simulink model "Static_Target_Final_2a"  (R2020b)
settings: Solver=FixedStepDiscrete  StartTime=0.0  StopTime=60*2  FixedStep=dt  RelTol=1e-3
InitFcn:
  | close all
  | clear
  | clc
  | 
  | dtsim = 0.1;
  | dt =0.005;
  | dtdata = 0.01;
  | dtcontrol = 0.01;
  | 
  | % Enviromental Constants/System Parameters
  | 
  | mu = 398600; %km^3/s^2 (Earth)
  | 
  | I = [1.01560749 0.00028915 0.00002257;
  |        0.00028915 0.17343628 0.00936307;
  |        0.00002257 0.00936307 1.01561864];
  | 
  | I_inv =[1/I(1,1) 0 0; 0 1/I(2,2) 0; 0 0 1/I(3,3)];
  | 
  | % Inital Conditions
  | 
  | Y = 0;
  | P = 0;
  | R = 0;
  | 
  | a = 6378;
  | n = sqrt(mu/a^3);
  | 
  | wo = [0;0;0];
  | ho = [0;0;0];
  | 
  | % YPR to Quaternion
  | 
  | qo = [-cos(R/2)*sin(P/2)*sin(Y/2) + sin(R/2)*cos(P/2)*cos(Y/2);
  |           cos(R/2)*sin(P/2)*cos(Y/2) + sin(R/2)*cos(P/2)*sin(Y/2);
  |          -sin(R/2)*sin(P/2)*cos(Y/2) + cos(R/2)*cos(P/2)*sin(Y/2);
  |           sin(R/2)*sin(P/2)*sin(Y/2) + cos(R/2)*cos(P/2)*cos(Y/2)];
  | 
  | % Reaction Wheels
  | 
  | x = cosd(70);
  | y = sqrt(0.5*(1^2-x^2));
  | e1 = [x;y;y];
  | e2 = [x;-y;y];
  | e3 = [x;-y;-y];
  | e4 = [x;y;-y];
  | %e1 = [y;x;y];
  | %e2 = [-y;x;y];
  | %e3 = [-y;-x;y];
  | %e4 = [y;-x;y];
  | e = [e1 e2 e3 e4];
  | 
  | % Reaction Wheels MOI and Ang Vel
  | 
  | Irw = 0.000453158;
  | 
  | w1 =1500*2*pi/60;
  | w2 = 1500*2*pi/60;
  | w3 = -1500*2*pi/60;
  | w4 = -1500*2*pi/60;
  | 
  | alpha_max = 1537.9; %rad/sec^2 Look at picture
  | 
  | Tmax = Irw*alpha_max; % Irw*alpha_max;
  | 
  | %User Input
  | 
  | Yt = 90*pi/180;
  | Pt = 10*pi/180;
  | Rt = 30*pi/180;
  | 
  | YPRtarget = [Yt, Pt, Rt];
  | 
  | %User Input Check
  | 
  | if Pt > 20*pi/180
  | 
  | error('Input a pitch angle lower that 20 degrees')
  | 
  | end
  | 
  | q_target = [-cos(Rt/2)*sin(Pt/2)*sin(Yt/2) + sin(Rt/2)*cos(Pt/2)*cos(Yt/2);
  |                   cos(Rt/2)*sin(Pt/2)*cos(Yt/2) + sin(Rt/2)*cos(Pt/2)*sin(Yt/2);
  |                  -sin(Rt/2)*sin(Pt/2)*cos(Yt/2) + cos(Rt/2)*cos(Pt/2)*sin(Yt/2);
  |                   sin(Rt/2)*sin(Pt/2)*sin(Yt/2) + cos(Rt/2)*cos(Pt/2)*cos(Yt/2)];
  | 
  | %LQR Controller
  | 
  | k1 = (I(2,2) - I(3,3))/I(1,1);
  | k2 = (I(2,2) - I(3,3))/I(2,2);
  | k3 = (I(2,2) - I(1,1))/I(3,3);
  | 
  | F = -2*n^2*[4*k1, 0, 0;0, 3*k2, 0; 0, 0, k3];
  | G = n*[0 0 (1-k1);0 0 0;(k3-1) 0 0 ];
  | 
  | A = [zeros(3,3) 0.5*eye(3);F G];
  | B = [zeros(3,3); I_inv];
  | R = eye(3);
  | R_inv = R^-1;
  | 
  | Q_nominal= diag([1,1,1,10,10,10]);
  | S_nominal = icare(A,B,Q_nominal,R);
  | K_nominal = -R_inv*B'*S_nominal;
  | 
  | Q_corrective= diag([1,1,1,10,10,10]);
  | S_corrective = icare(A,B,Q_corrective,R);
  | K_corrective = -R_inv*B'*S_corrective;
  | 
  | Q_yawsweep= diag([1,1,1,10,15,10]);
  | S_yawsweep = icare(A,B,Q_yawsweep,R);
  | K_yawsweep = -R_inv*B'*S_yawsweep;
  | 
  | % Visual Int
  | 
  | myworld = vrworld('SimulinkTest.wrl');
  | open(myworld);
  | 
  | set(0,'Units','pixels');
  | scnsize = get(0,'ScreenSize');
  | 
  | f1 = vrfigure(myworld,scnsize);
StopFcn:
  | close all
  | 
  | %Set default grid axes to be on
  | set(groot,'defaultAxesXGrid','on')
  | set(groot,'defaultAxesYGrid','on')
  | 
  | 
  | %Create YPR subplots
  | figure(1)
  | subplot(1,3,1)
  | movegui('northeast')
  | plot(YPR.time,YPR.signals.values(:,1)*180/pi,'-k')
  | hold on
  | plot([0 YPR.time(end)], [1,1]*(rad2deg(YPRtarget(1))+1),'-r')
  | plot([0 YPR.time(end)], [1,1]*(rad2deg(YPRtarget(1))-1),'-r')
  | xlabel('Time (s)')
  | ylabel('Roll (deg)')
  | xlim([0 YPR.time(end)])
  | 
  | set(gca, 'FontSize', 15)
  | 
  | subplot(1,3,2)
  | plot(YPR.time,YPR.signals.values(:,2)*180/pi,'-k')
  | hold on
  | plot([0 YPR.time(end)],  [1,1]*(rad2deg(YPRtarget(2))+1),'-r')
  | plot([0 YPR.time(end)], [1,1]*(rad2deg(YPRtarget(2))-1),'-r')
  | xlabel('Time (s)')
  | ylabel('Pitch (deg)')
  | xlim([0 YPR.time(end)])
  | 
  | set(gca, 'FontSize', 15)
  | 
  | subplot(1,3,3)
  | plot(YPR.time,YPR.signals.values(:,3)*180/pi,'-k')
  | hold on
  | plot([0 YPR.time(end)],  [1,1]*(rad2deg(YPRtarget(3))+1),'-r')
  | plot([0 YPR.time(end)], [1,1]*(rad2deg(YPRtarget(3))-1),'-r')
  | xlabel('Time (s)')
  | ylabel('Yaw (deg)')
  | xlim([0 YPR.time(end)])
  | 
  | set(gca, 'FontSize', 15)
  | 
  | 
  | %Create Angular Position Plots
  | 
  | MagnitudeAngle = 2*acos(q_target(1))*180/pi;
  | 
  | figure(2)
  | movegui('northwest')
  | 
  | hold on
  | 
  | plot(YPR.time,YPR_Mag,'-k')
  | plot([0 YPR.time(end)],  [1,1]*(MagnitudeAngle+1),'-r')
  | plot([0 YPR.time(end)], [1,1]*(MagnitudeAngle-1),'-r')
  | xlabel('Time (sec)')
  | ylabel('Angle (deg)')
  | xlim([0 YPR.time(end)])
  | title('Angular Position Magnitude')
  | box on
  | 
  | 
  | % Create Motor Torque plot
  | figure(3)
  | movegui('south')
  | 
  | %plot(YPR.time,(Motor_Torques.signals.values(1,:)/Tmax)*100,YPR.time,(Motor_Torques.signals.values(2,:)/Tmax)*100,YPR.time,(Motor_Torques.signals.values(3,:)/Tmax)*100,YPR.time,(Motor_Torques.signals.values(4,:)/Tmax)*100)
  | plot(YPR.time,Motor_Torques.signals.values(1,:),YPR.time,Motor_Torques.signals.values(2,:),YPR.time,Motor_Torques.signals.values(3,:),YPR.time,Motor_Torques.signals.values(4,:))
  | xlabel('Time (s)')
  | %ylabel('Torque Percentage (%)')
  | ylabel('Torque (Nm)')
  | title('Motor Torques')
  | legend('Top Motor','Right Motor','Left Motor','Bottom Motor')
  | 
  | 
  | %Create Angular Speed plot
  | figure(4)
  | movegui('southwest')
  | 
  | wmag = sqrt(wvec.signals.values(1,:).^2+wvec.signals.values(2,:).^2+wvec.signals.values(3,:).^2)*180/pi;
  | hold on
  | plot(YPR.time,wmag)
  | plot(YPR.time,0.25.*ones(numel(YPR.time),1))
  | %plot(YPR.time,60*ones(numel(YPR.time),1))
  | xlabel('Time (s)')
  | ylabel('Angular Speed (deg/s)')
  | ylim([-0.5, 20])
  | xlim([0 YPR.time(end)])
  | title('Angular Speed Magnitude')
  | legend('System Angluar Speed', '0.25 deg/s')
  | grid on
  | 
  | 
  | %Create YPR Error plot
  | figure(5)
  | movegui('southeast')
  | hold on
  | plot(YPRerror.time(:,1)', YPRerror.signals.values(:,1), YPRerror.time(:,1)', YPRerror.signals.values(:,2), YPRerror.time(:,1)', YPRerror.signals.values(:,3))
  | plot(YPRerror.time(:,1)', zeros(length(YPRerror.time),1), '--')
  | xlabel('Time (s)')
  | ylabel('Error (°)')
  | title('YPR Error')
  | legend('Roll Error', 'Pitch Error', 'Yaw Error', 'Zero Error')
  | 
  | 
  | %Create Controller Type plot
  | figure(6)
  | movegui('north')
  | 
  | plot(controllerMode.time(:,1)', controllerMode.signals.values)
  | xlabel('Time (s)')
  | ylabel('Controller ID Tag')
  | title('LQR Control Mode vs Time')
  | ylim([0 4])
  | yticks([1,2,3])
undefined symbols (not defined in the file): DiscIntNeverNeededParam
libraries: vrlib x2, dspinverses x1, simulink x1
settings Model: Creator=lewisbreslin  LastModifiedBy=bnich
settings DataIOCC: ReturnWorkspaceOutputs=off
settings DebuggingCC: ArithmeticOperatorsInVariantConditions=warning
settings SFSimCC: SimUseLocalCustomCode=off  CustomCodeUndefinedFunction=UseInterfaceOnly
settings RTWCC: RTWUseLocalCustomCode=off
settings CodeAppCC: StateflowObjectComments=on

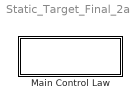
== system Static_Target_Final_2a ==
  "Main Control Law " : Subsystem  TreatAsAtomicUnit=on

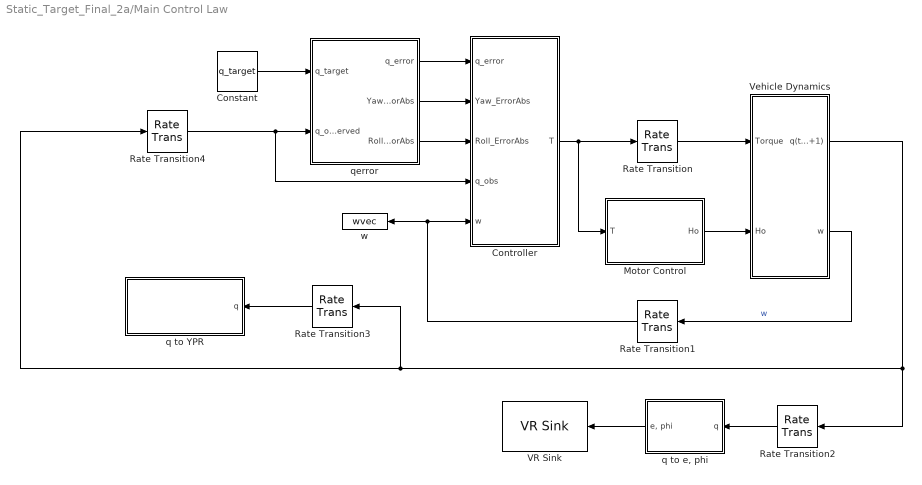
== system Static_Target_Final_2a/Main Control Law  ==
  Constant : Constant  Value=q_target
  Controller : Subsystem
  Motor Control : Subsystem
  Rate Transition : RateTransition  OutPortSampleTime=dt
  Rate Transition1 : RateTransition  InitialCondition=wo  OutPortSampleTime=dtcontrol
  Rate Transition2 : RateTransition  InitialCondition=qo  OutPortSampleTime=dtsim
  Rate Transition3 : RateTransition  InitialCondition=qo  OutPortSampleTime=dtdata
  Rate Transition4 : RateTransition  InitialCondition=qo  OutPortSampleTime=dtcontrol
  VR Sink : vrlib/VR Sink  InstantiateOnLoad=on  SampleTime=0.1  ViewEnable=on  RemoteChange=off  RemoteView=off  FieldsWritten=Phoenix.rotation.4.1.1.double  WorldFileName=SimulinkTest.wrl  AutoView=off  VideoDimensions=[]  AllowVariableSize=off
  Vehicle Dynamics : Subsystem
  q to YPR : Subsystem  TreatAsAtomicUnit=on
  "q to e, phi " : Subsystem
  qerror : Subsystem
  "w " : ToWorkspace  VariableName=wvec  SaveFormat=Structure With Time  SampleTime=-1
  wires:
  Vehicle Dynamics/2(w) -> Rate Transition1/1  "w"
  Controller/1(T) -> Rate Transition/1, Motor Control/1(T)
  Motor Control/1(Ho) -> Vehicle Dynamics/2("Ho ")
  qerror/3(Roll_ErrorAbs) -> Controller/3(Roll_ErrorAbs)
  Rate Transition3/1 -> q to YPR/1(q)
  qerror/2(Yaw_ErrorAbs) -> Controller/2(Yaw_ErrorAbs)
  qerror/1(q_error) -> Controller/1(q_error)
  Rate Transition2/1 -> "q to e, phi "/1(q)
  Constant/1 -> qerror/1(q_target)
  Rate Transition1/1 -> Controller/5(w), "w "/1
  Vehicle Dynamics/1(q(t_k+1)) -> Rate Transition2/1, Rate Transition4/1, Rate Transition3/1
  Rate Transition/1 -> Vehicle Dynamics/1(Torque)
  Rate Transition4/1 -> Controller/4(q_obs), qerror/2(q_observed)
  "q to e, phi "/1("e, phi") -> VR Sink/1

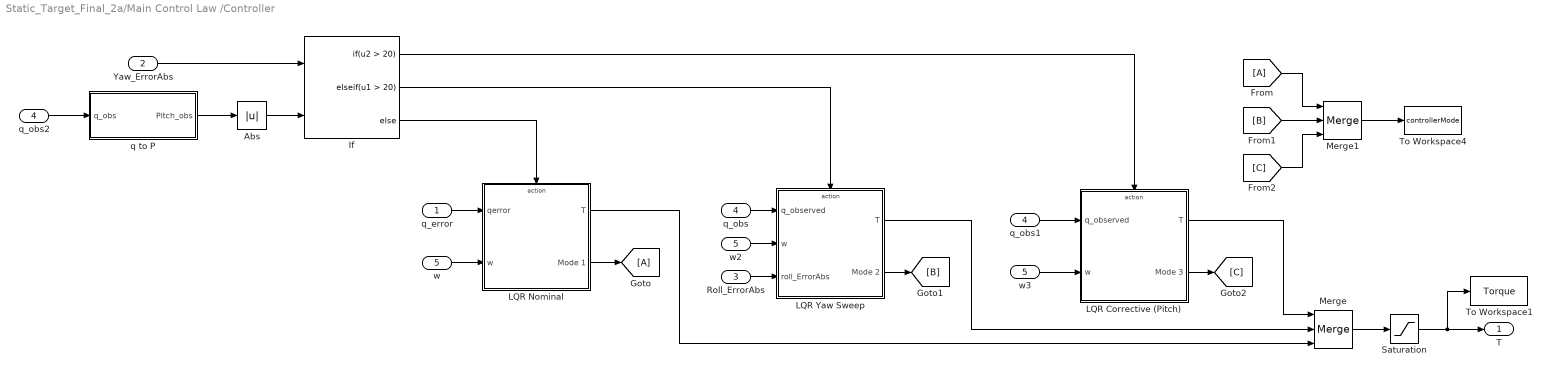
== system Static_Target_Final_2a/Main Control Law /Controller ==
  q_error : Inport
  Yaw_ErrorAbs : Inport  Port=2
  Roll_ErrorAbs : Inport  Port=3
  q_obs : Inport  Port=4
  w : Inport  Port=5
  Abs : Abs
  If : If  NumInputs=2  IfExpression=u2 > 20  ElseIfExpressions=u1 > 20
  LQR Corrective (Pitch) : Subsystem
  LQR Nominal : Subsystem  TreatAsAtomicUnit=on
  LQR Yaw Sweep : Subsystem
  Merge : Merge  Inputs=3
  Merge1 : Merge  Inputs=3
  Saturation : Saturate  UpperLimit=Tmax  LowerLimit=-Tmax
  To Workspace1 : ToWorkspace  VariableName=Torque  SaveFormat=Structure With Time  SampleTime=-1
  To Workspace4 : ToWorkspace  VariableName=controllerMode  SaveFormat=Structure With Time  SampleTime=-1
  q to P : Subsystem
  q_obs1 : InportShadow  Port=4
  q_obs2 : InportShadow  Port=4
  w2 : InportShadow  Port=5
  w3 : InportShadow  Port=5
  T : Outport
  wires:
  Yaw_ErrorAbs/1 -> If/1
  If/3 -> LQR Nominal/Action
  q_error/1 -> LQR Nominal/1(qerror)
  If/1 -> LQR Corrective (Pitch)/Action
  q_obs1/1 -> LQR Corrective (Pitch)/1(q_observed)
  q_obs/1 -> LQR Yaw Sweep/1(q_observed)
  q to P/1(Pitch_obs) -> Abs/1
  If/2 -> LQR Yaw Sweep/Action
  LQR Nominal/2(Mode 1) -> [A]
  LQR Yaw Sweep/2(Mode 2) -> [B]
  LQR Corrective (Pitch)/2(Mode 3) -> [C]
  [B] -> Merge1/2
  [A] -> Merge1/1
  [C] -> Merge1/3
  Merge1/1 -> To Workspace4/1
  w3/1 -> LQR Corrective (Pitch)/2(w)
  w2/1 -> LQR Yaw Sweep/2(w)
  w/1 -> LQR Nominal/2(w)
  q_obs2/1 -> q to P/1(q_obs)
  Abs/1 -> If/2
  Roll_ErrorAbs/1 -> LQR Yaw Sweep/3(roll_ErrorAbs)
  LQR Nominal/1(T) -> Merge/3
  LQR Yaw Sweep/1(T) -> Merge/2
  LQR Corrective (Pitch)/1(T) -> Merge/1
  Merge/1 -> Saturation/1
  Saturation/1 -> To Workspace1/1, T/1

== system Static_Target_Final_2a/Main Control Law /Motor Control ==
  T : Inport
  Actuator : Subsystem
  Motor control : Subsystem
  Ho : Outport
  wires:
  T/1 -> Actuator/1(Torque)
  Actuator/2(alpha_RW) -> Motor control/2(alpha_RW)
  Motor control/1(Ho) -> Ho/1
  Actuator/1(Irw*e) -> Motor control/1(Irw*e)

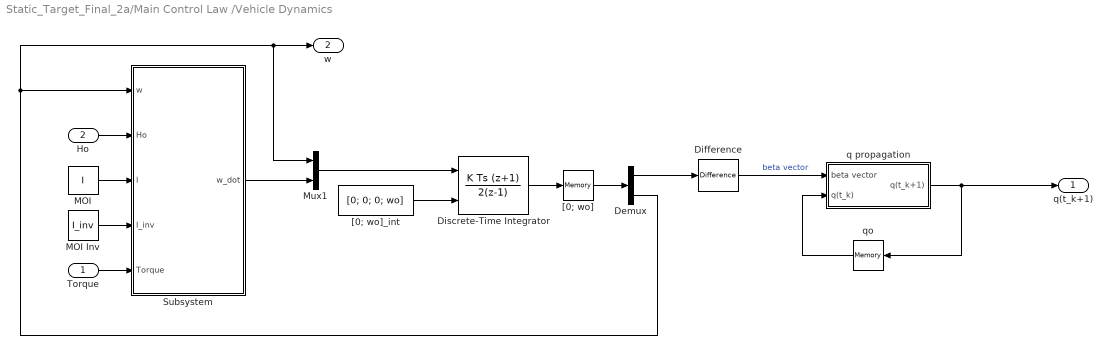
== system Static_Target_Final_2a/Main Control Law /Vehicle Dynamics ==
  Torque : Inport
  "Ho " : Inport  Port=2
  Demux : Demux  Outputs=2
  Difference : simulink/Discrete/Difference  ICPrevInput=[0;0;0]  OutMin=[]  OutMax=[]  OutDataType=fixdt(1, 16)  OutScaling=2^-10  DoSatur=off
  Discrete-Time Integrator : DiscreteIntegrator  IntegratorMethod=Integration: Trapezoidal  InitialConditionSource=external  SampleTime=dt  ICPrevOutput=DiscIntNeverNeededParam  ICPrevScaledInput=DiscIntNeverNeededParam
  MOI : Constant  Value=I
  MOI Inv : Constant  Value=I_inv
  Mux1 : Mux  Inputs=2
  Subsystem : Subsystem
  "[0; wo]" : Memory  InitialCondition=[0;0;0;wo]  InheritSampleTime=on
  "[0; wo]_int" : Constant  Value=[0; 0; 0; wo]  VectorParams1D=off  SampleTime=dt
  q propagation : Subsystem
  qo : Memory  InitialCondition=qo  InheritSampleTime=on
  q(t_k+1) : Outport
  w : Outport  Port=2
  wires:
  "Ho "/1 -> Subsystem/2("Ho ")
  Torque/1 -> Subsystem/5(Torque)
  MOI Inv/1 -> Subsystem/4(I_inv)
  MOI/1 -> Subsystem/3(I)
  Subsystem/1(w_dot) -> Mux1/2
  Difference/1 -> q propagation/1("beta vector ")  "beta vector"
  "[0; wo]_int"/1 -> Discrete-Time Integrator/2
  q propagation/1(q(t_k+1)) -> q(t_k+1)/1, qo/1
  qo/1 -> q propagation/2(q(t_k))
  Demux/1 -> Difference/1
  Discrete-Time Integrator/1 -> "[0; wo]"/1
  "[0; wo]"/1 -> Demux/1
  Mux1/1 -> Discrete-Time Integrator/1
  Demux/2 -> w/1, Mux1/1, Subsystem/1(w)

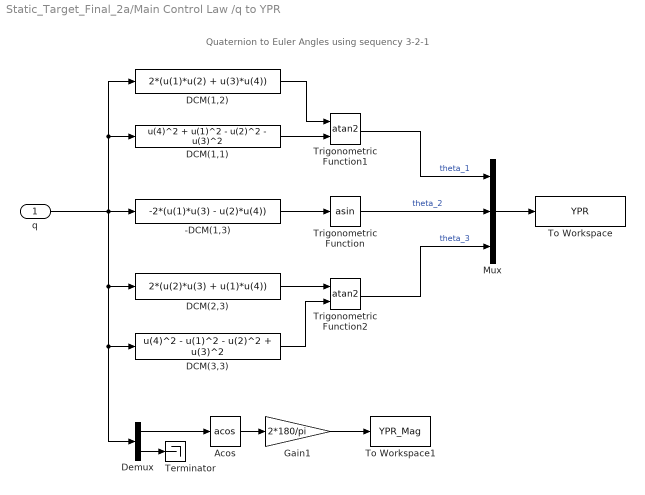
== system Static_Target_Final_2a/Main Control Law /q to YPR ==
  note: Quaternion to Euler Angles using sequency 3-2-1
  q : Inport
  -DCM(1,3) : Fcn  Expr=-2*(u(1)*u(3) - u(2)*u(4))
  Acos : Trigonometry  Operator=acos
  DCM(1,1) : Fcn  Expr=u(4)^2 + u(1)^2 - u(2)^2 - u(3)^2
  DCM(1,2) : Fcn  Expr=2*(u(1)*u(2) + u(3)*u(4))
  DCM(2,3) : Fcn  Expr=2*(u(2)*u(3) + u(1)*u(4))
  DCM(3,3) : Fcn  Expr=u(4)^2 - u(1)^2 - u(2)^2 + u(3)^2
  Demux : Demux  Outputs=[1;3]
  Gain1 : Gain  Gain=2*180/pi
  Mux : Mux  Inputs=3
  Terminator : Terminator
  To Workspace : ToWorkspace  VariableName=YPR  SaveFormat=Structure With Time  SampleTime=dtdata
  To Workspace1 : ToWorkspace  VariableName=YPR_Mag  SampleTime=dtdata
  Trigonometric Function : Trigonometry  Operator=asin
  Trigonometric Function1 : Trigonometry  Operator=atan2
  Trigonometric Function2 : Trigonometry  Operator=atan2
  wires:
  q/1 -> Demux/1, DCM(3,3)/1, DCM(2,3)/1, -DCM(1,3)/1, DCM(1,2)/1, DCM(1,1)/1
  -DCM(1,3)/1 -> Trigonometric Function/1
  DCM(2,3)/1 -> Trigonometric Function2/1
  DCM(1,2)/1 -> Trigonometric Function1/1
  DCM(1,1)/1 -> Trigonometric Function1/2
  DCM(3,3)/1 -> Trigonometric Function2/2
  Trigonometric Function/1 -> Mux/2  "theta_2"
  Trigonometric Function2/1 -> Mux/3  "theta_3"
  Trigonometric Function1/1 -> Mux/1  "theta_1"
  Mux/1 -> To Workspace/1
  Gain1/1 -> To Workspace1/1
  Acos/1 -> Gain1/1
  Demux/1 -> Acos/1
  Demux/2 -> Terminator/1

== system Static_Target_Final_2a/Main Control Law /q to e, phi  ==
  note: Quaternion to Euler Angles using sequency 3-2-1
  q : Inport
  Demux : Demux  Outputs=[3, 1]
  Divide : Product  Inputs=*/
  Gain : Gain  Gain=2
  Mux : Mux  Inputs=2
  Trigonometric Function : Trigonometry  Operator=acos
  Trigonometric Function1 : Trigonometry
  "e, phi" : Outport
  wires:
  Gain/1 -> Mux/2  "phi"
  Demux/2 -> Trigonometric Function/1  "q4"
  Trigonometric Function/1 -> Gain/1, Trigonometric Function1/1  "phi/2"
  Demux/1 -> Divide/1  "q_hat"
  Divide/1 -> Mux/1  "e"
  Trigonometric Function1/1 -> Divide/2  "sin(phi/2)"
  Mux/1 -> "e, phi"/1
  q/1 -> Demux/1

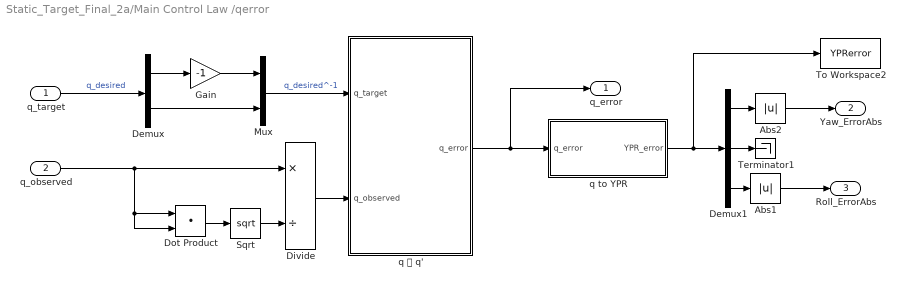
== system Static_Target_Final_2a/Main Control Law /qerror ==
  q_target : Inport
  q_observed : Inport  Port=2
  Abs1 : Abs
  Abs2 : Abs
  Demux : Demux  Outputs=[3,1]
  Demux1 : Demux  Outputs=3
  Divide : Product  Inputs=*/
  Dot Product : DotProduct  InputSameDT=on  OutDataTypeStr=Inherit: Inherit via internal rule
  Gain : Gain  Gain=-1
  Mux : Mux  Inputs=2
  Sqrt : Sqrt  SaturateOnIntegerOverflow=on
  Terminator1 : Terminator
  To Workspace2 : ToWorkspace  VariableName=YPRerror  SaveFormat=Structure With Time  SampleTime=-1
  q to YPR : Subsystem  TreatAsAtomicUnit=on
  q ⦻ q' : Subsystem  TreatAsAtomicUnit=on
  q_error : Outport
  Yaw_ErrorAbs : Outport  Port=2
  Roll_ErrorAbs : Outport  Port=3
  wires:
  Abs2/1 -> Yaw_ErrorAbs/1
  Demux1/2 -> Terminator1/1
  Abs1/1 -> Roll_ErrorAbs/1
  Divide/1 -> q ⦻ q'/2(q_observed)
  q_observed/1 -> Divide/1, Dot Product/1, Dot Product/2
  Dot Product/1 -> Sqrt/1
  q ⦻ q'/1(q_error) -> q to YPR/1(q_error), q_error/1
  Gain/1 -> Mux/1
  Mux/1 -> q ⦻ q'/1(q_target)  "q_desired^-1"
  q_target/1 -> Demux/1  "q_desired"
  Demux/1 -> Gain/1
  Sqrt/1 -> Divide/2
  Demux/2 -> Mux/2
  q to YPR/1(YPR_error) -> Demux1/1, To Workspace2/1
  Demux1/1 -> Abs2/1
  Demux1/3 -> Abs1/1

== system Static_Target_Final_2a/Main Control Law /Controller/LQR Corrective (Pitch) ==
  q_observed : Inport
  w : Inport  Port=2
  Action Port : ActionPort  ActionPortLabel=if(u2 > 20)
  Constant : Constant  Value=3
  LQR Corrective (Pitch) : Subsystem
  q_adjustment : Subsystem
  q_error : Subsystem
  T : Outport
  Mode 3 : Outport  Port=2
  wires:
  Constant/1 -> Mode 3/1
  LQR Corrective (Pitch)/1(T) -> T/1
  w/1 -> LQR Corrective (Pitch)/2(w)
  q_adjustment/1(q_adjusted) -> q_error/1(q_target)
  q_observed/1 -> q_adjustment/1(q_obs), q_error/2(q_observed)
  q_error/1(q_error) -> LQR Corrective (Pitch)/1(q_error)

== system Static_Target_Final_2a/Main Control Law /Controller/LQR Nominal ==
  qerror : Inport
  w : Inport  Port=2
  Action Port : ActionPort  ActionPortLabel=else
  Constant : Constant
  LQR Nominal : Subsystem
  T : Outport
  Mode 1 : Outport  Port=2
  wires:
  Constant/1 -> Mode 1/1
  qerror/1 -> LQR Nominal/1(q_error)
  LQR Nominal/1(T) -> T/1
  w/1 -> LQR Nominal/2(w)

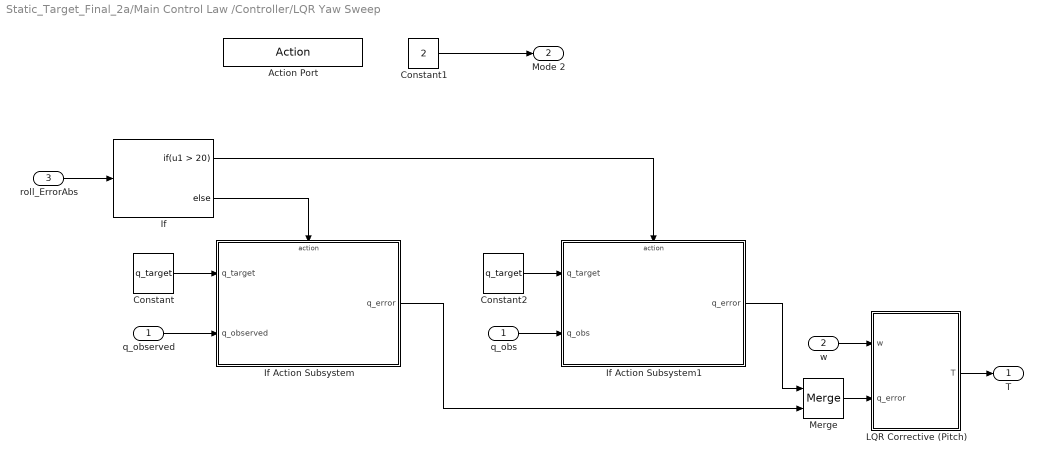
== system Static_Target_Final_2a/Main Control Law /Controller/LQR Yaw Sweep ==
  q_observed : Inport
  w : Inport  Port=2
  roll_ErrorAbs : Inport  Port=3
  Action Port : ActionPort  ActionPortLabel=elseif(u1 > 20)
  Constant : Constant  Value=q_target
  Constant1 : Constant  Value=2
  Constant2 : Constant  Value=q_target
  If : If  IfExpression=u1 > 20
  If Action Subsystem : Subsystem  TreatAsAtomicUnit=on
  If Action Subsystem1 : Subsystem  TreatAsAtomicUnit=on
  LQR Corrective (Pitch) : Subsystem
  Merge : Merge
  q_obs : InportShadow
  T : Outport
  Mode 2 : Outport  Port=2
  wires:
  roll_ErrorAbs/1 -> If/1
  Constant/1 -> If Action Subsystem/1(q_target)
  Constant1/1 -> Mode 2/1
  If/2 -> If Action Subsystem/Action
  LQR Corrective (Pitch)/1(T) -> T/1
  w/1 -> LQR Corrective (Pitch)/1(w)
  If/1 -> If Action Subsystem1/Action
  q_observed/1 -> If Action Subsystem/2(q_observed)
  Merge/1 -> LQR Corrective (Pitch)/2(q_error)
  If Action Subsystem1/1(q_error) -> Merge/1
  If Action Subsystem/1(q_error) -> Merge/2
  q_obs/1 -> If Action Subsystem1/2(q_obs)
  Constant2/1 -> If Action Subsystem1/1(q_target)

== system Static_Target_Final_2a/Main Control Law /Controller/q to P ==
  q_obs : Inport
  -DCM(1,3) : Fcn  Expr=-2*(u(1)*u(3) - u(2)*u(4))
  Gain2 : Gain  Gain=180/pi
  Trigonometric Function1 : Trigonometry  Operator=asin
  Pitch_obs : Outport
  wires:
  Gain2/1 -> Pitch_obs/1
  Trigonometric Function1/1 -> Gain2/1  "P"
  -DCM(1,3)/1 -> Trigonometric Function1/1
  q_obs/1 -> -DCM(1,3)/1

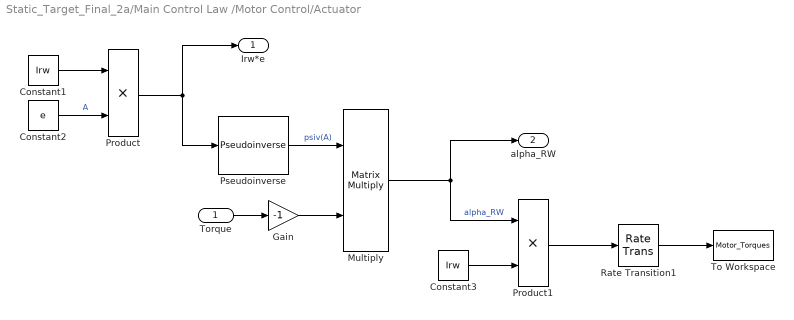
== system Static_Target_Final_2a/Main Control Law /Motor Control/Actuator ==
  Torque : Inport  PortDimensions=[3,1]
  Constant1 : Constant  Value=Irw
  Constant2 : Constant  Value=e
  Constant3 : Constant  Value=Irw
  Gain : Gain  Gain=-1
  Multiply : Product  Multiplication=Matrix(*)
  Product : Product
  Product1 : Product
  Pseudoinverse : dspinverses/Pseudoinverse  wanterr=off  SimulateUsing=Interpreted execution
      settings: SourceProductBaseCode=DS
  Rate Transition1 : RateTransition  InitialCondition=[0;0;0;0]  OutPortSampleTime=dtdata
  To Workspace : ToWorkspace  VariableName=Motor_Torques  SaveFormat=Structure With Time  SampleTime=dtdata
  Irw*e : Outport
  alpha_RW : Outport  Port=2
  wires:
  Torque/1 -> Gain/1
  Product/1 -> Irw*e/1, Pseudoinverse/1
  Constant1/1 -> Product/1
  Pseudoinverse/1 -> Multiply/1  "psiv(A)"
  Multiply/1 -> Product1/1, alpha_RW/1  "alpha_RW"
  Constant2/1 -> Product/2  "A"
  Gain/1 -> Multiply/2
  Constant3/1 -> Product1/2
  Product1/1 -> Rate Transition1/1
  Rate Transition1/1 -> To Workspace/1

== system Static_Target_Final_2a/Main Control Law /Motor Control/Motor control ==
  Irw*e : Inport
  alpha_RW : Inport  Port=2
  Constant3 : Constant  Value=[w1 ;w2 ;w3 ;w4]  SampleTime=dt
  Discrete-Time Integrator1 : DiscreteIntegrator  IntegratorMethod=Integration: Trapezoidal  InitialConditionSource=external  SampleTime=dt  LimitOutput=on  UpperSaturationLimit=733  LowerSaturationLimit=-733  ICPrevOutput=DiscIntNeverNeededParam  ICPrevScaledInput=DiscIntNeverNeededParam
  Multiply3 : Product  Multiplication=Matrix(*)
  Ho : Outport
  wires:
  Irw*e/1 -> Multiply3/1  "Irw*e"
  Constant3/1 -> Discrete-Time Integrator1/2
  Multiply3/1 -> Ho/1
  Discrete-Time Integrator1/1 -> Multiply3/2
  alpha_RW/1 -> Discrete-Time Integrator1/1

== system Static_Target_Final_2a/Main Control Law /Vehicle Dynamics/Subsystem ==
  note: $\dot{\bar{\omega}}=[I]^{-1}\left(\bar{T}-\bar{\omega} \times\left([I]\bar{\omega}+\bar{H_0}\right)\right)$
  w : Inport
  "Ho " : Inport  Port=2
  I : Inport  Port=3
  I_inv : Inport  Port=4
  Torque : Inport  Port=5
  Add1 : Sum  Inputs=|++
  Cross Product : vrlib/Utilities/Cross Product
  Matrix Multiply2 : Product  Multiplication=Matrix(*)
  Matrix Multiply3 : Product  Multiplication=Matrix(*)
  Sum : Sum  Inputs=|+-
  w_dot : Outport
  wires:
  I/1 -> Matrix Multiply2/1
  w/1 -> Cross Product/1, Matrix Multiply2/2
  Torque/1 -> Sum/1
  Sum/1 -> Matrix Multiply3/2
  Cross Product/1 -> Sum/2
  Matrix Multiply3/1 -> w_dot/1
  I_inv/1 -> Matrix Multiply3/1
  Matrix Multiply2/1 -> Add1/1
  Add1/1 -> Cross Product/2
  "Ho "/1 -> Add1/2

== system Static_Target_Final_2a/Main Control Law /Vehicle Dynamics/q propagation ==
  "beta vector " : Inport
  q(t_k) : Inport  Port=2
  Dot Product : DotProduct  InputSameDT=on  OutDataTypeStr=Inherit: Inherit via internal rule
  Sqrt : Sqrt  SaturateOnIntegerOverflow=on
  if/esle condition : Subsystem
  q * q' : Subsystem  TreatAsAtomicUnit=on
  q(t_k+1) : Outport
  wires:
  "beta vector "/1 -> Dot Product/2, Dot Product/1, if/esle condition/1("beta vector ")
  if/esle condition/1(q') -> q * q'/2(q')
  q(t_k)/1 -> q * q'/1(q)
  q * q'/1(q'') -> q(t_k+1)/1
  Dot Product/1 -> Sqrt/1
  Sqrt/1 -> if/esle condition/2(norm(beta))

== system Static_Target_Final_2a/Main Control Law /qerror/q to YPR ==
  note: Quaternion to Euler Angles using sequency 3-2-1
  q_error : Inport
  -DCM(1,3) : Fcn  Expr=-2*(u(1)*u(3) - u(2)*u(4))
  DCM(1,1) : Fcn  Expr=u(4)^2 + u(1)^2 - u(2)^2 - u(3)^2
  DCM(1,2) : Fcn  Expr=2*(u(1)*u(2) + u(3)*u(4))
  DCM(2,3) : Fcn  Expr=2*(u(2)*u(3) + u(1)*u(4))
  DCM(3,3) : Fcn  Expr=u(4)^2 - u(1)^2 - u(2)^2 + u(3)^2
  Gain2 : Gain  Gain=180/pi
  Mux : Mux  Inputs=3
  Trigonometric Function : Trigonometry  Operator=asin
  Trigonometric Function1 : Trigonometry  Operator=atan2
  Trigonometric Function2 : Trigonometry  Operator=atan2
  YPR_error : Outport
  wires:
  q_error/1 -> DCM(3,3)/1, DCM(2,3)/1, -DCM(1,3)/1, DCM(1,2)/1, DCM(1,1)/1
  -DCM(1,3)/1 -> Trigonometric Function/1
  DCM(2,3)/1 -> Trigonometric Function2/1
  DCM(1,2)/1 -> Trigonometric Function1/1
  DCM(1,1)/1 -> Trigonometric Function1/2
  DCM(3,3)/1 -> Trigonometric Function2/2
  Trigonometric Function/1 -> Mux/2  "P"
  Trigonometric Function2/1 -> Mux/3  "R"
  Trigonometric Function1/1 -> Mux/1  "Y"
  Gain2/1 -> YPR_error/1
  Mux/1 -> Gain2/1

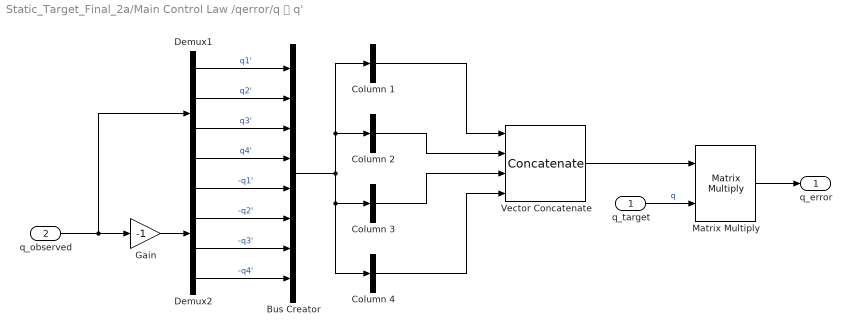
== system Static_Target_Final_2a/Main Control Law /qerror/q ⦻ q' ==
  q_target : Inport
  q_observed : Inport  Port=2
  Bus Creator : BusCreator  Inputs=8
  Column 1 : BusSelector  OutputSignals=q4',-q3',q2',-q1'  OutputAsBus=on
  Column 2 : BusSelector  OutputSignals=q3',q4',-q1',-q2'  OutputAsBus=on
  Column 3 : BusSelector  OutputSignals=-q2',q1',q4',-q3'  OutputAsBus=on
  Column 4 : BusSelector  OutputSignals=q1',q2',q3',q4'  OutputAsBus=on
  Demux1 : Demux
  Demux2 : Demux
  Gain : Gain  Gain=-1
  Matrix Multiply : Product  Multiplication=Matrix(*)
  Vector Concatenate : Concatenate  NumInputs=4  Mode=Multidimensional array  ConcatenateDimension=2
  q_error : Outport
  wires:
  Gain/1 -> Demux2/1
  Demux1/1 -> Bus Creator/1  "q1'"
  Demux1/3 -> Bus Creator/3  "q3'"
  Demux1/2 -> Bus Creator/2  "q2'"
  Demux2/4 -> Bus Creator/8  "-q4'"
  Demux2/3 -> Bus Creator/7  "-q3'"
  Demux2/2 -> Bus Creator/6  "-q2'"
  Demux2/1 -> Bus Creator/5  "-q1'"
  Demux1/4 -> Bus Creator/4  "q4'"
  Bus Creator/1 -> Column 4/1, Column 3/1, Column 1/1, Column 2/1
  Column 1/1 -> Vector Concatenate/1
  Column 2/1 -> Vector Concatenate/2
  Column 3/1 -> Vector Concatenate/3
  Column 4/1 -> Vector Concatenate/4
  q_observed/1 -> Demux1/1, Gain/1
  q_target/1 -> Matrix Multiply/2  "q"
  Matrix Multiply/1 -> q_error/1
  Vector Concatenate/1 -> Matrix Multiply/1

== system Static_Target_Final_2a/Main Control Law /Controller/LQR Corrective (Pitch)/LQR Corrective (Pitch) ==
  q_error : Inport
  w : Inport  Port=2
  Constant3 : Constant  Value=K_corrective
  Demux1 : Demux  Outputs=[3,1]
  Mux1 : Mux  Inputs=2
  Product : Product  Multiplication=Matrix(*)
  Terminator1 : Terminator
  T : Outport
  wires:
  Product/1 -> T/1
  q_error/1 -> Demux1/1
  Constant3/1 -> Product/1
  Demux1/1 -> Mux1/1  "qhat_Error"
  w/1 -> Mux1/2
  Mux1/1 -> Product/2  "xbar"
  Demux1/2 -> Terminator1/1

== system Static_Target_Final_2a/Main Control Law /Controller/LQR Corrective (Pitch)/q_adjustment ==
  q_obs : Inport
  DCM(1,1) : Fcn  Expr=u(4)^2 + u(1)^2 - u(2)^2 - u(3)^2
  DCM(1,2) : Fcn  Expr=2*(u(1)*u(2) + u(3)*u(4))
  DCM(2,3) : Fcn  Expr=2*(u(2)*u(3) + u(1)*u(4))
  DCM(3,3) : Fcn  Expr=u(4)^2 - u(1)^2 - u(2)^2 + u(3)^2
  Trigonometric Function4 : Trigonometry  Operator=atan2
  Trigonometric Function5 : Trigonometry  Operator=atan2
  YPR to q : Subsystem
  q_adjusted : Outport
  wires:
  Trigonometric Function5/1 -> YPR to q/2(R)  "R"
  DCM(2,3)/1 -> Trigonometric Function5/1
  DCM(1,1)/1 -> Trigonometric Function4/2
  DCM(3,3)/1 -> Trigonometric Function5/2
  DCM(1,2)/1 -> Trigonometric Function4/1
  q_obs/1 -> DCM(3,3)/1, DCM(2,3)/1, DCM(1,2)/1, DCM(1,1)/1
  YPR to q/1(q_adjusted) -> q_adjusted/1
  Trigonometric Function4/1 -> YPR to q/1(Y)  "Y"

== system Static_Target_Final_2a/Main Control Law /Controller/LQR Corrective (Pitch)/q_error ==
  q_target : Inport
  q_observed : Inport  Port=2
  Demux : Demux  Outputs=[3,1]
  Divide : Product  Inputs=*/
  Dot Product : DotProduct  InputSameDT=on  OutDataTypeStr=Inherit: Inherit via internal rule
  Gain : Gain  Gain=-1
  Mux : Mux  Inputs=2
  Sqrt : Sqrt  SaturateOnIntegerOverflow=on
  q ⦻ q' : Subsystem  TreatAsAtomicUnit=on
  q_error : Outport
  wires:
  q ⦻ q'/1(q_error) -> q_error/1
  Mux/1 -> q ⦻ q'/1(q_target)  "q_desired^-1"
  Sqrt/1 -> Divide/2
  Demux/1 -> Gain/1
  q_target/1 -> Demux/1  "q_desired"
  Gain/1 -> Mux/1
  q_observed/1 -> Divide/1, Dot Product/1, Dot Product/2
  Dot Product/1 -> Sqrt/1
  Demux/2 -> Mux/2
  Divide/1 -> q ⦻ q'/2(q_observed)

== system Static_Target_Final_2a/Main Control Law /Controller/LQR Nominal/LQR Nominal ==
  q_error : Inport
  w : Inport  Port=2
  Constant3 : Constant  Value=K_nominal
  Demux1 : Demux  Outputs=[3,1]
  Mux1 : Mux  Inputs=2
  Product : Product  Multiplication=Matrix(*)
  Terminator1 : Terminator
  T : Outport
  wires:
  Mux1/1 -> Product/2  "xbar"
  Demux1/1 -> Mux1/1  "qhat_Error"
  q_error/1 -> Demux1/1
  Demux1/2 -> Terminator1/1
  w/1 -> Mux1/2
  Constant3/1 -> Product/1
  Product/1 -> T/1

== system Static_Target_Final_2a/Main Control Law /Controller/LQR Yaw Sweep/If Action Subsystem ==
  q_target : Inport
  q_observed : Inport  Port=2
  Action Port : ActionPort  ActionPortLabel=else
  q_adjustment : Subsystem
  qerror : Subsystem
  q_error : Outport
  wires:
  q_target/1 -> q_adjustment/1(q_target)
  qerror/1(q_error) -> q_error/1
  q_observed/1 -> qerror/2(q_observed)
  q_adjustment/1(q_adjusted) -> qerror/1(q_target)

== system Static_Target_Final_2a/Main Control Law /Controller/LQR Yaw Sweep/If Action Subsystem1 ==
  q_target : Inport
  q_obs : Inport  Port=2
  Action Port : ActionPort  ActionPortLabel=if(u1 > 20)
  q_adjustment : Subsystem
  qerror : Subsystem
  q_error : Outport
  wires:
  q_adjustment/1(q_adjusted) -> qerror/1(q_target)
  q_target/1 -> q_adjustment/1(q_target)
  q_obs/1 -> qerror/2(q_observed), q_adjustment/2(q_obs)
  qerror/1(q_error) -> q_error/1

== system Static_Target_Final_2a/Main Control Law /Controller/LQR Yaw Sweep/LQR Corrective (Pitch) ==
  w : Inport
  q_error : Inport  Port=2
  Constant3 : Constant  Value=K_yawsweep
  Demux1 : Demux  Outputs=[3,1]
  Mux1 : Mux  Inputs=2
  Product : Product  Multiplication=Matrix(*)
  Terminator1 : Terminator
  T : Outport
  wires:
  Product/1 -> T/1
  q_error/1 -> Demux1/1
  Constant3/1 -> Product/1
  Demux1/1 -> Mux1/1  "qhat_Error"
  w/1 -> Mux1/2
  Mux1/1 -> Product/2  "xbar"
  Demux1/2 -> Terminator1/1

== system Static_Target_Final_2a/Main Control Law /Vehicle Dynamics/q propagation/if//esle condition ==
  "beta vector " : Inport
  norm(beta) : Inport  Port=2
  If : If  IfExpression=u1 < 1e-10
  If Action Subsystem : Subsystem  TreatAsAtomicUnit=on
  If Action Subsystem1 : Subsystem  TreatAsAtomicUnit=on
  Merge : Merge
  q' : Outport
  wires:
  If Action Subsystem/1(q') -> Merge/1
  Merge/1 -> q'/1
  If Action Subsystem1/1(q') -> Merge/2
  If/2 -> If Action Subsystem1/Action
  norm(beta)/1 -> If Action Subsystem1/1(norm(beta)), If/1
  If/1 -> If Action Subsystem/Action
  "beta vector "/1 -> If Action Subsystem1/2("beta vector ")

== system Static_Target_Final_2a/Main Control Law /Vehicle Dynamics/q propagation/q * q' ==
  q : Inport
  q' : Inport  Port=2
  Bus Creator : BusCreator  Inputs=8
  Column 1 : BusSelector  OutputSignals=q4',-q3',q2',-q1'  OutputAsBus=on
  Column 2 : BusSelector  OutputSignals=q3',q4',-q1',-q2'  OutputAsBus=on
  Column 3 : BusSelector  OutputSignals=-q2',q1',q4',-q3'  OutputAsBus=on
  Column 4 : BusSelector  OutputSignals=q1',q2',q3',q4'  OutputAsBus=on
  Demux1 : Demux
  Demux2 : Demux
  Gain : Gain  Gain=-1
  Matrix Multiply : Product  Multiplication=Matrix(*)
  Vector Concatenate : Concatenate  NumInputs=4  Mode=Multidimensional array  ConcatenateDimension=2
  q'' : Outport
  wires:
  Gain/1 -> Demux2/1
  Demux1/1 -> Bus Creator/1  "q1'"
  Demux1/3 -> Bus Creator/3  "q3'"
  Demux1/2 -> Bus Creator/2  "q2'"
  Demux2/4 -> Bus Creator/8  "-q4'"
  Demux2/3 -> Bus Creator/7  "-q3'"
  Demux2/2 -> Bus Creator/6  "-q2'"
  Demux2/1 -> Bus Creator/5  "-q1'"
  Demux1/4 -> Bus Creator/4  "q4'"
  Bus Creator/1 -> Column 4/1, Column 3/1, Column 1/1, Column 2/1
  Column 1/1 -> Vector Concatenate/1
  Column 2/1 -> Vector Concatenate/2
  Column 3/1 -> Vector Concatenate/3
  Column 4/1 -> Vector Concatenate/4
  q'/1 -> Demux1/1, Gain/1
  q/1 -> Matrix Multiply/2  "q"
  Matrix Multiply/1 -> q''/1
  Vector Concatenate/1 -> Matrix Multiply/1

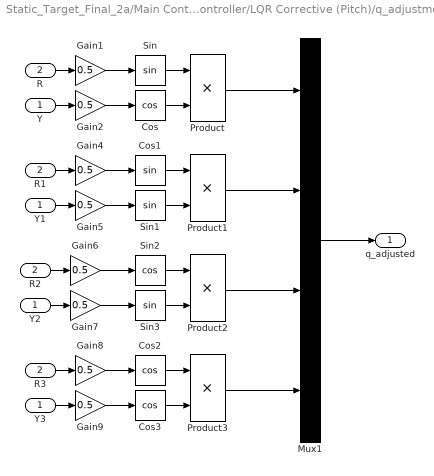
== system Static_Target_Final_2a/Main Control Law /Controller/LQR Corrective (Pitch)/q_adjustment/YPR to q ==
  Y : Inport
  R : Inport  Port=2
  Cos : Trigonometry  Operator=cos
  Cos1 : Trigonometry
  Cos2 : Trigonometry  Operator=cos
  Cos3 : Trigonometry  Operator=cos
  Gain{1..2,4..9} (8 alike) : Gain  Gain=0.5
  Mux1 : Mux
  Product{,1..3} (4 alike) : Product
  R1 : InportShadow  Port=2
  R2 : InportShadow  Port=2
  R3 : InportShadow  Port=2
  Sin : Trigonometry
  Sin1 : Trigonometry
  Sin2 : Trigonometry  Operator=cos
  Sin3 : Trigonometry
  Y1 : InportShadow
  Y2 : InportShadow
  Y3 : InportShadow
  q_adjusted : Outport
  wires:
  Gain2/1 -> Cos/1
  Sin/1 -> Product/1
  Sin3/1 -> Product2/2
  Sin1/1 -> Product1/2
  Mux1/1 -> q_adjusted/1
  Cos/1 -> Product/2
  Sin2/1 -> Product2/1
  Gain8/1 -> Cos2/1
  Cos1/1 -> Product1/1
  Gain6/1 -> Sin2/1
  Product3/1 -> Mux1/4
  Product/1 -> Mux1/1
  Gain5/1 -> Sin1/1
  Gain9/1 -> Cos3/1
  Gain4/1 -> Cos1/1
  Cos2/1 -> Product3/1
  Product1/1 -> Mux1/2
  Gain7/1 -> Sin3/1
  Gain1/1 -> Sin/1
  Cos3/1 -> Product3/2
  R1/1 -> Gain4/1
  Y1/1 -> Gain5/1
  R2/1 -> Gain6/1
  Y2/1 -> Gain7/1
  Y3/1 -> Gain9/1
  R3/1 -> Gain8/1
  Y/1 -> Gain2/1
  R/1 -> Gain1/1
  Product2/1 -> Mux1/3

== system Static_Target_Final_2a/Main Control Law /Controller/LQR Corrective (Pitch)/q_error/q ⦻ q' ==
  q_target : Inport
  q_observed : Inport  Port=2
  Bus Creator : BusCreator  Inputs=8
  Column 1 : BusSelector  OutputSignals=q4',-q3',q2',-q1'  OutputAsBus=on
  Column 2 : BusSelector  OutputSignals=q3',q4',-q1',-q2'  OutputAsBus=on
  Column 3 : BusSelector  OutputSignals=-q2',q1',q4',-q3'  OutputAsBus=on
  Column 4 : BusSelector  OutputSignals=q1',q2',q3',q4'  OutputAsBus=on
  Demux1 : Demux
  Demux2 : Demux
  Gain : Gain  Gain=-1
  Matrix Multiply : Product  Multiplication=Matrix(*)
  Vector Concatenate : Concatenate  NumInputs=4  Mode=Multidimensional array  ConcatenateDimension=2
  q_error : Outport
  wires:
  Gain/1 -> Demux2/1
  Demux1/1 -> Bus Creator/1  "q1'"
  Demux1/3 -> Bus Creator/3  "q3'"
  Demux1/2 -> Bus Creator/2  "q2'"
  Demux2/4 -> Bus Creator/8  "-q4'"
  Demux2/3 -> Bus Creator/7  "-q3'"
  Demux2/2 -> Bus Creator/6  "-q2'"
  Demux2/1 -> Bus Creator/5  "-q1'"
  Demux1/4 -> Bus Creator/4  "q4'"
  Bus Creator/1 -> Column 4/1, Column 3/1, Column 1/1, Column 2/1
  Column 1/1 -> Vector Concatenate/1
  Column 2/1 -> Vector Concatenate/2
  Column 3/1 -> Vector Concatenate/3
  Column 4/1 -> Vector Concatenate/4
  q_observed/1 -> Demux1/1, Gain/1
  q_target/1 -> Matrix Multiply/2  "q"
  Matrix Multiply/1 -> q_error/1
  Vector Concatenate/1 -> Matrix Multiply/1

== system Static_Target_Final_2a/Main Control Law /Controller/LQR Yaw Sweep/If Action Subsystem/q_adjustment ==
  q_target : Inport
  DCM(1,1) : Fcn  Expr=u(4)^2 + u(1)^2 - u(2)^2 - u(3)^2
  DCM(1,2) : Fcn  Expr=2*(u(1)*u(2) + u(3)*u(4))
  DCM(2,3) : Fcn  Expr=2*(u(2)*u(3) + u(1)*u(4))
  DCM(3,3) : Fcn  Expr=u(4)^2 - u(1)^2 - u(2)^2 + u(3)^2
  Trigonometric Function4 : Trigonometry  Operator=atan2
  Trigonometric Function5 : Trigonometry  Operator=atan2
  YPR to q : Subsystem
  q_adjusted : Outport
  wires:
  YPR to q/1(q_adjusted) -> q_adjusted/1
  Trigonometric Function5/1 -> YPR to q/2(R)  "R"
  DCM(3,3)/1 -> Trigonometric Function5/2
  DCM(1,1)/1 -> Trigonometric Function4/2
  DCM(2,3)/1 -> Trigonometric Function5/1
  Trigonometric Function4/1 -> YPR to q/1(Y)  "Y"
  DCM(1,2)/1 -> Trigonometric Function4/1
  q_target/1 -> DCM(3,3)/1, DCM(2,3)/1, DCM(1,2)/1, DCM(1,1)/1

== system Static_Target_Final_2a/Main Control Law /Controller/LQR Yaw Sweep/If Action Subsystem/qerror ==
  q_target : Inport
  q_observed : Inport  Port=2
  Demux : Demux  Outputs=[3,1]
  Divide : Product  Inputs=*/
  Dot Product : DotProduct  InputSameDT=on  OutDataTypeStr=Inherit: Inherit via internal rule
  Gain : Gain  Gain=-1
  Mux : Mux  Inputs=2
  Sqrt : Sqrt  SaturateOnIntegerOverflow=on
  q ⦻ q' : Subsystem  TreatAsAtomicUnit=on
  q_error : Outport
  wires:
  Sqrt/1 -> Divide/2
  Dot Product/1 -> Sqrt/1
  Gain/1 -> Mux/1
  Mux/1 -> q ⦻ q'/1(q_target)  "q_desired^-1"
  q ⦻ q'/1(q_error) -> q_error/1
  q_observed/1 -> Divide/1, Dot Product/1, Dot Product/2
  q_target/1 -> Demux/1  "q_desired"
  Demux/1 -> Gain/1
  Demux/2 -> Mux/2
  Divide/1 -> q ⦻ q'/2(q_observed)

== system Static_Target_Final_2a/Main Control Law /Controller/LQR Yaw Sweep/If Action Subsystem1/q_adjustment ==
  q_target : Inport
  q_obs : Inport  Port=2
  DCM(1,1) : Fcn  Expr=u(4)^2 + u(1)^2 - u(2)^2 - u(3)^2
  DCM(1,2) : Fcn  Expr=2*(u(1)*u(2) + u(3)*u(4))
  DCM(2,3) : Fcn  Expr=2*(u(2)*u(3) + u(1)*u(4))
  DCM(3,3) : Fcn  Expr=u(4)^2 - u(1)^2 - u(2)^2 + u(3)^2
  Trigonometric Function4 : Trigonometry  Operator=atan2
  Trigonometric Function5 : Trigonometry  Operator=atan2
  YPR to q : Subsystem
  q_adjusted : Outport
  wires:
  YPR to q/1(q_adjusted) -> q_adjusted/1
  Trigonometric Function5/1 -> YPR to q/2(R)  "R"
  DCM(1,1)/1 -> Trigonometric Function4/2
  DCM(3,3)/1 -> Trigonometric Function5/2
  DCM(1,2)/1 -> Trigonometric Function4/1
  DCM(2,3)/1 -> Trigonometric Function5/1
  Trigonometric Function4/1 -> YPR to q/1(Y)  "Y"
  q_target/1 -> DCM(1,1)/1, DCM(1,2)/1
  q_obs/1 -> DCM(2,3)/1, DCM(3,3)/1

== system Static_Target_Final_2a/Main Control Law /Controller/LQR Yaw Sweep/If Action Subsystem1/qerror ==
  q_target : Inport
  q_observed : Inport  Port=2
  Demux : Demux  Outputs=[3,1]
  Divide : Product  Inputs=*/
  Dot Product : DotProduct  InputSameDT=on  OutDataTypeStr=Inherit: Inherit via internal rule
  Gain : Gain  Gain=-1
  Mux : Mux  Inputs=2
  Sqrt : Sqrt  SaturateOnIntegerOverflow=on
  q ⦻ q' : Subsystem  TreatAsAtomicUnit=on
  q_error : Outport
  wires:
  q ⦻ q'/1(q_error) -> q_error/1
  Mux/1 -> q ⦻ q'/1(q_target)  "q_desired^-1"
  Sqrt/1 -> Divide/2
  Demux/1 -> Gain/1
  q_target/1 -> Demux/1  "q_desired"
  Gain/1 -> Mux/1
  q_observed/1 -> Divide/1, Dot Product/1, Dot Product/2
  Dot Product/1 -> Sqrt/1
  Demux/2 -> Mux/2
  Divide/1 -> q ⦻ q'/2(q_observed)

== system Static_Target_Final_2a/Main Control Law /Vehicle Dynamics/q propagation/if//esle condition/If Action Subsystem ==
  Action Port : ActionPort  ActionPortLabel=if(u1 < 1e-10)
  Constant : Constant  Value=[0;0;0;1]  VectorParams1D=off  SampleTime=dt
  q' : Outport
  wires:
  Constant/1 -> q'/1

== system Static_Target_Final_2a/Main Control Law /Vehicle Dynamics/q propagation/if//esle condition/If Action Subsystem1 ==
  norm(beta) : Inport
  "beta vector " : Inport  Port=2
  Action Port : ActionPort  ActionPortLabel=else
  Cos : Trigonometry  Operator=cos
  Divide : Product  Inputs=*/
  Gain : Gain  Gain=0.5
  Multiply : Product  Inputs=**
  Sin : Trigonometry
  Vector Concatenate : Concatenate
  q' : Outport
  wires:
  Cos/1 -> Vector Concatenate/2
  Divide/1 -> Multiply/1
  Sin/1 -> Multiply/2
  Vector Concatenate/1 -> q'/1
  Multiply/1 -> Vector Concatenate/1
  norm(beta)/1 -> Divide/2, Gain/1
  Gain/1 -> Cos/1, Sin/1  "norm(beta)/2"
  "beta vector "/1 -> Divide/1

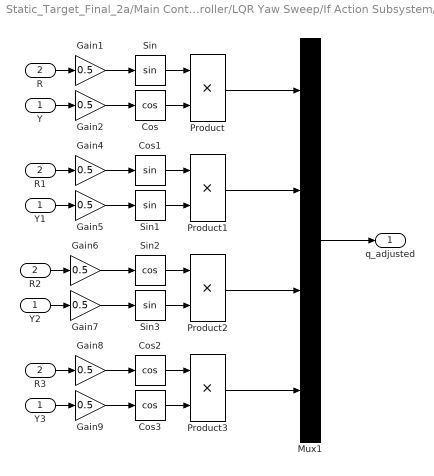
== system Static_Target_Final_2a/Main Control Law /Controller/LQR Yaw Sweep/If Action Subsystem/q_adjustment/YPR to q ==
  Y : Inport
  R : Inport  Port=2
  Cos : Trigonometry  Operator=cos
  Cos1 : Trigonometry
  Cos2 : Trigonometry  Operator=cos
  Cos3 : Trigonometry  Operator=cos
  Gain{1..2,4..9} (8 alike) : Gain  Gain=0.5
  Mux1 : Mux
  Product{,1..3} (4 alike) : Product
  R1 : InportShadow  Port=2
  R2 : InportShadow  Port=2
  R3 : InportShadow  Port=2
  Sin : Trigonometry
  Sin1 : Trigonometry
  Sin2 : Trigonometry  Operator=cos
  Sin3 : Trigonometry
  Y1 : InportShadow
  Y2 : InportShadow
  Y3 : InportShadow
  q_adjusted : Outport
  wires:
  Gain2/1 -> Cos/1
  Sin/1 -> Product/1
  Sin3/1 -> Product2/2
  Sin1/1 -> Product1/2
  Mux1/1 -> q_adjusted/1
  Cos/1 -> Product/2
  Sin2/1 -> Product2/1
  Gain8/1 -> Cos2/1
  Cos1/1 -> Product1/1
  Gain6/1 -> Sin2/1
  Product3/1 -> Mux1/4
  Product/1 -> Mux1/1
  Gain5/1 -> Sin1/1
  Gain9/1 -> Cos3/1
  Gain4/1 -> Cos1/1
  Cos2/1 -> Product3/1
  Product1/1 -> Mux1/2
  Gain7/1 -> Sin3/1
  Gain1/1 -> Sin/1
  Cos3/1 -> Product3/2
  R1/1 -> Gain4/1
  Y1/1 -> Gain5/1
  R2/1 -> Gain6/1
  Y2/1 -> Gain7/1
  Y3/1 -> Gain9/1
  R3/1 -> Gain8/1
  Y/1 -> Gain2/1
  R/1 -> Gain1/1
  Product2/1 -> Mux1/3

== system Static_Target_Final_2a/Main Control Law /Controller/LQR Yaw Sweep/If Action Subsystem/qerror/q ⦻ q' ==
  q_target : Inport
  q_observed : Inport  Port=2
  Bus Creator : BusCreator  Inputs=8
  Column 1 : BusSelector  OutputSignals=q4',-q3',q2',-q1'  OutputAsBus=on
  Column 2 : BusSelector  OutputSignals=q3',q4',-q1',-q2'  OutputAsBus=on
  Column 3 : BusSelector  OutputSignals=-q2',q1',q4',-q3'  OutputAsBus=on
  Column 4 : BusSelector  OutputSignals=q1',q2',q3',q4'  OutputAsBus=on
  Demux1 : Demux
  Demux2 : Demux
  Gain : Gain  Gain=-1
  Matrix Multiply : Product  Multiplication=Matrix(*)
  Vector Concatenate : Concatenate  NumInputs=4  Mode=Multidimensional array  ConcatenateDimension=2
  q_error : Outport
  wires:
  Gain/1 -> Demux2/1
  Demux1/1 -> Bus Creator/1  "q1'"
  Demux1/3 -> Bus Creator/3  "q3'"
  Demux1/2 -> Bus Creator/2  "q2'"
  Demux2/4 -> Bus Creator/8  "-q4'"
  Demux2/3 -> Bus Creator/7  "-q3'"
  Demux2/2 -> Bus Creator/6  "-q2'"
  Demux2/1 -> Bus Creator/5  "-q1'"
  Demux1/4 -> Bus Creator/4  "q4'"
  Bus Creator/1 -> Column 4/1, Column 3/1, Column 1/1, Column 2/1
  Column 1/1 -> Vector Concatenate/1
  Column 2/1 -> Vector Concatenate/2
  Column 3/1 -> Vector Concatenate/3
  Column 4/1 -> Vector Concatenate/4
  q_observed/1 -> Demux1/1, Gain/1
  q_target/1 -> Matrix Multiply/2  "q"
  Matrix Multiply/1 -> q_error/1
  Vector Concatenate/1 -> Matrix Multiply/1

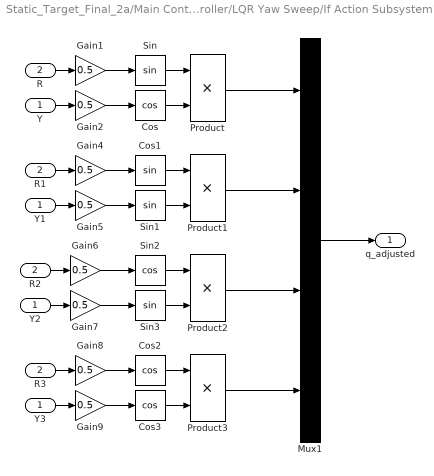
== system Static_Target_Final_2a/Main Control Law /Controller/LQR Yaw Sweep/If Action Subsystem1/q_adjustment/YPR to q ==
  Y : Inport
  R : Inport  Port=2
  Cos : Trigonometry  Operator=cos
  Cos1 : Trigonometry
  Cos2 : Trigonometry  Operator=cos
  Cos3 : Trigonometry  Operator=cos
  Gain{1..2,4..9} (8 alike) : Gain  Gain=0.5
  Mux1 : Mux
  Product{,1..3} (4 alike) : Product
  R1 : InportShadow  Port=2
  R2 : InportShadow  Port=2
  R3 : InportShadow  Port=2
  Sin : Trigonometry
  Sin1 : Trigonometry
  Sin2 : Trigonometry  Operator=cos
  Sin3 : Trigonometry
  Y1 : InportShadow
  Y2 : InportShadow
  Y3 : InportShadow
  q_adjusted : Outport
  wires:
  Gain2/1 -> Cos/1
  Sin/1 -> Product/1
  Sin3/1 -> Product2/2
  Sin1/1 -> Product1/2
  Mux1/1 -> q_adjusted/1
  Cos/1 -> Product/2
  Sin2/1 -> Product2/1
  Gain8/1 -> Cos2/1
  Cos1/1 -> Product1/1
  Gain6/1 -> Sin2/1
  Product3/1 -> Mux1/4
  Product/1 -> Mux1/1
  Gain5/1 -> Sin1/1
  Gain9/1 -> Cos3/1
  Gain4/1 -> Cos1/1
  Cos2/1 -> Product3/1
  Product1/1 -> Mux1/2
  Gain7/1 -> Sin3/1
  Gain1/1 -> Sin/1
  Cos3/1 -> Product3/2
  R1/1 -> Gain4/1
  Y1/1 -> Gain5/1
  R2/1 -> Gain6/1
  Y2/1 -> Gain7/1
  Y3/1 -> Gain9/1
  R3/1 -> Gain8/1
  Y/1 -> Gain2/1
  R/1 -> Gain1/1
  Product2/1 -> Mux1/3

== system Static_Target_Final_2a/Main Control Law /Controller/LQR Yaw Sweep/If Action Subsystem1/qerror/q ⦻ q' ==
  q_target : Inport
  q_observed : Inport  Port=2
  Bus Creator : BusCreator  Inputs=8
  Column 1 : BusSelector  OutputSignals=q4',-q3',q2',-q1'  OutputAsBus=on
  Column 2 : BusSelector  OutputSignals=q3',q4',-q1',-q2'  OutputAsBus=on
  Column 3 : BusSelector  OutputSignals=-q2',q1',q4',-q3'  OutputAsBus=on
  Column 4 : BusSelector  OutputSignals=q1',q2',q3',q4'  OutputAsBus=on
  Demux1 : Demux
  Demux2 : Demux
  Gain : Gain  Gain=-1
  Matrix Multiply : Product  Multiplication=Matrix(*)
  Vector Concatenate : Concatenate  NumInputs=4  Mode=Multidimensional array  ConcatenateDimension=2
  q_error : Outport
  wires:
  Gain/1 -> Demux2/1
  Demux1/1 -> Bus Creator/1  "q1'"
  Demux1/3 -> Bus Creator/3  "q3'"
  Demux1/2 -> Bus Creator/2  "q2'"
  Demux2/4 -> Bus Creator/8  "-q4'"
  Demux2/3 -> Bus Creator/7  "-q3'"
  Demux2/2 -> Bus Creator/6  "-q2'"
  Demux2/1 -> Bus Creator/5  "-q1'"
  Demux1/4 -> Bus Creator/4  "q4'"
  Bus Creator/1 -> Column 4/1, Column 3/1, Column 1/1, Column 2/1
  Column 1/1 -> Vector Concatenate/1
  Column 2/1 -> Vector Concatenate/2
  Column 3/1 -> Vector Concatenate/3
  Column 4/1 -> Vector Concatenate/4
  q_observed/1 -> Demux1/1, Gain/1
  q_target/1 -> Matrix Multiply/2  "q"
  Matrix Multiply/1 -> q_error/1
  Vector Concatenate/1 -> Matrix Multiply/1
